simulink model "elevator2"  (Simulink 6.5)
settings: Solver=FixedStepDiscrete  StartTime=0.0  StopTime=inf  FixedStep=0.01  RelTol=1e-3
libraries: simulink x2
settings Model: Creator=sja  LastModifiedBy=haf  ExtModeAutoUpdateStatusClock=off
settings DebuggingCC: MultiTaskDSMMsg=warning  MultiTaskCondExecSysMsg=none  StrictBusMsg=None
settings RTWCC: IncludeERTFirstTime=on

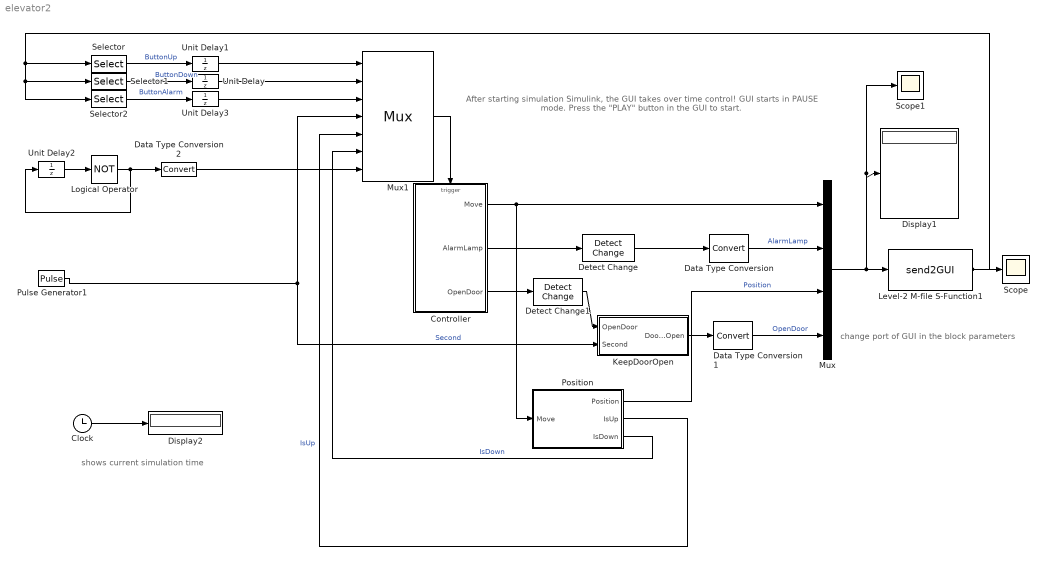
== system elevator2 ==
  note: change port of
      | GUI in the block
      | parameters
  note: shows current simulation time
  note: After starting simulation Simulink, the GUI takes over time control!
      | GUI starts in PAUSE mode.
      | Press the "PLAY" button in the GUI to start.
  Clock : Clock
      settings: Decimation=10
  Controller : Stateflow chart
  Data Type Conversion : DataTypeConversion
  Data Type Conversion1 : DataTypeConversion
  Data Type Conversion2 : DataTypeConversion  OutDataTypeMode=double
  Detect Change : simulink/Logic and Bit Operations/Detect Change  SystemSampleTime=-1  vinit=0
  Detect Change1 : simulink/Logic and Bit Operations/Detect Change  SystemSampleTime=-1  vinit=0
  Display1 : Display
  Display2 : Display
      settings: Decimation=3
  KeepDoorOpen : Subsystem
  Level-2 M-file S-Function1 : M-S-Function  FunctionName=send2GUI  Parameters=port,dimensions,sampletime  mask{port=1234, dimensions=3, sampletime=-1}
      mask prompts: port "TCP Port for GUI server"; dimensions "Output Port Dimensions"
      mask help: Interface Block to pass data between the model and a graphical user interface accessed via TCP/IP.
      mask Display:
      | fprintf('GUI INTERFACE\n\n')
      | fprintf(['Port: ' num2str(port)])
  Logical Operator : Logic  Operator=NOT  OutDataTypeMode=Boolean  LogicDataType=double
  Mux : Mux
  Mux1 : Mux  Inputs=7
      settings: DisplayOption=signals
  Position : Subsystem
  Pulse Generator1 : DiscretePulseGenerator  PulseType=Time based  Amplitude=2  Period=6  PulseWidth=50
  Scope : Scope
      settings: YMin=0.95  YMax=1.05
  Scope1 : Scope
      settings: YMin=0.95  YMax=1.05
  Selector : Selector  InputType=Vector  ElementSrc=Internal  Elements=1  RowSrc=Internal  Rows=1  ColumnSrc=Internal  Columns=1  IndexIsStartValue=off
  Selector1 : Selector  InputType=Vector  ElementSrc=Internal  Elements=2  RowSrc=Internal  Rows=1  ColumnSrc=Internal  Columns=1  IndexIsStartValue=off
  Selector2 : Selector  InputType=Vector  ElementSrc=Internal  Elements=3  RowSrc=Internal  Rows=1  ColumnSrc=Internal  Columns=1  IndexIsStartValue=off
  Unit Delay{,1..3} (4 alike) : UnitDelay  SampleTime=-1
  wires:
  Mux/1 -> Display1/1, Scope1/1, Level-2 M-file S-Function1/1
  Level-2 M-file S-Function1/1 -> Scope/1, Selector/1, Selector1/1, Selector2/1
  Controller/1(Move) -> Position/1(Move), Mux/1
  Controller/2(AlarmLamp) -> Detect Change/1
  Mux1/1 -> Controller/Trigger
  Pulse Generator1/1 -> Mux1/4, KeepDoorOpen/2(Second)  "Second"
  Data Type Conversion/1 -> Mux/2  "AlarmLamp"
  Position/1(Position) -> Mux/3  "Position"
  Position/2(IsUp) -> Mux1/5  "IsUp"
  Position/3(IsDown) -> Mux1/6  "IsDown"
  Data Type Conversion1/1 -> Mux/4  "OpenDoor"
  KeepDoorOpen/1(DoorIsOpen) -> Data Type Conversion1/1
  Controller/3(OpenDoor) -> Detect Change1/1
  Selector/1 -> Unit Delay1/1  "ButtonUp"
  Selector2/1 -> Unit Delay3/1  "ButtonAlarm"
  Selector1/1 -> Unit Delay/1  "ButtonDown"
  Unit Delay1/1 -> Mux1/1
  Unit Delay/1 -> Mux1/2
  Unit Delay3/1 -> Mux1/3
  Unit Delay2/1 -> Logical Operator/1
  Logical Operator/1 -> Unit Delay2/1, Data Type Conversion2/1
  Data Type Conversion2/1 -> Mux1/7
  Detect Change/1 -> Data Type Conversion/1
  Detect Change1/1 -> KeepDoorOpen/1(OpenDoor)
  Clock/1 -> Display2/1

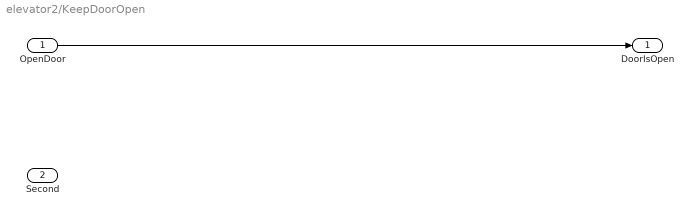
== system elevator2/KeepDoorOpen ==
  OpenDoor : Inport
  Second : Inport  Port=2
  DoorIsOpen : Outport
  wires:
  OpenDoor/1 -> DoorIsOpen/1

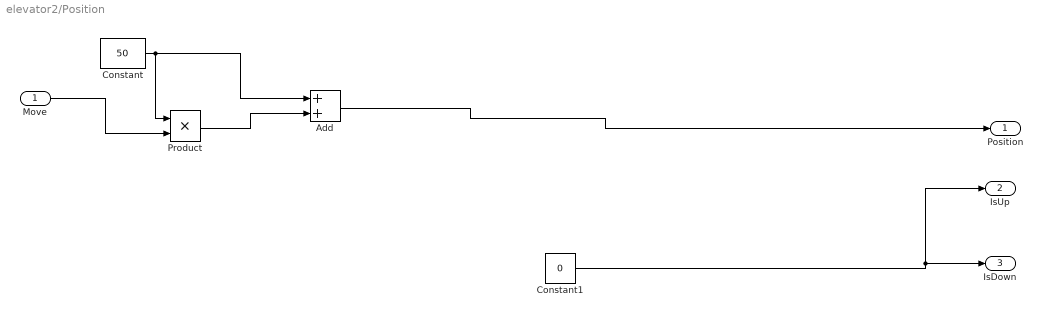
== system elevator2/Position ==
  Move : Inport
  Add : Sum  OutScaling=2^-10
  Constant : Constant  Value=50
  Constant1 : Constant  Value=0
  Product : Product  RndMeth=Zero
  Position : Outport
  IsUp : Outport  Port=2
  IsDown : Outport  Port=3
  wires:
  Add/1 -> Position/1
  Constant1/1 -> IsDown/1, IsUp/1
  Constant/1 -> Add/1, Product/1
  Product/1 -> Add/2
  Move/1 -> Product/2

== stateflow chart Controller ==
  state Normal
    state Down
    Down -> Down [order 1] : ButtonDown/Move:=-1,OpenDoor
    (default) -> Down
    Down -> Down [order 2] : ButtonUp/Move:=1, OpenDoor
  state Error
    du: AlarmLamp
  state Alarm
    state Off
    state On
      du: AlarmLamp
    (default) -> On
    On -> Off : Second
    Off -> On : Second
  Normal -> Error : ButtonAlarm / Move:=0
  Error -> (history) [order 2] : Second / Move:=-1
  Error -> Alarm [order 1] : ButtonAlarm
  (default) -> Normal
  data: Move output double; data local double; Dir local double
  events: ButtonUp input EITHER_EDGE_EVENT; ButtonDown input EITHER_EDGE_EVENT; ButtonAlarm input EITHER_EDGE_EVENT; AlarmLamp output EITHER_EDGE_EVENT; Second input RISING_EDGE_EVENT; IsUp input RISING_EDGE_EVENT; IsDown input RISING_EDGE_EVENT; OpenDoor output EITHER_EDGE_EVENT; Dummy input EITHER_EDGE_EVENT
